simulink model "single_phase_multilevel"  (R2023b)
settings: Solver=ode1be  StartTime=0.0  StopTime=simlength  FixedStep=tc  RelTol=1e-3
values from neighbouring files (symbols this model uses):
  Vfc1_base = Udc/5    [plotting_modulation.m]
  Vfc2_base = 2*Vfc1_base    [plotting_modulation.m]
  Vfc3_base = 3*Vfc1_base    [plotting_modulation.m]
  Vfc4_base = 4*Vfc1_base    [plotting_modulation.m]
undefined symbols (not defined in the file or in its folder): __PRM__SERIALIZED__DATA__, DThs_init, g0_4Hz, g1_4Hz, I_FS, kalman_omega, kalman_theta, ki_i_inv, ki_v_inv, kp_i_inv, kp_v_inv, Lconn, LFu1, m_dead_time, m_duty_open_loop, magnitude, n10, omega_ref, phase_shift_mod11, phase_shift_mod21, phase_shift_mod31, phase_shift_mod41, phase_shift_mod51, precharge_off, q1kalman, q2kalman, Rbalance, Rconn, RFu, Rg_off, Rg_on, Rkalman, RLFu1, Rprecharge, Tambient, tc, time_pwm_enable, tPWM, ts, V_FS, VCFc_5_init, Vgate_base, weigth
libraries: fl_lib x271, nesl_utility x97, ee_lib x15, simulink x1
(part 4 of 5)

== system single_phase_multilevel/flying_capacitor_leg/switch_51 ==
  G : Inport
  Current Sensor : fl_lib/Electrical/Electrical Sensors/Current Sensor
  Electrical Reference : fl_lib/Electrical/Electrical Elements/Electrical Reference
  G3R160MT17D : ee_lib/Semiconductors & Converters/MOSFET (Ideal, Switching)  port_option=ee.enum.controlport.elec  Rds=Rds_on Ohm  Goff=Goff_state_mosfet 1/Ohm  Vth=Vg_threshold V  diode_param=ee.enum.converters.protectiondiode.nodynamics  diode_Vf=Vgamma_diode_mosfet V  diode_Ron=Ron_diode_mosfet Ohm  diode_Goff=Goff_state_mosfet 1/Ohm  diode_C=50e-9 F  diode_iRM=-235 A  diode_iF=300 A  diode_idot=-50 A/us  diode_trr_param=ee.enum.converters.diodeReverseParam.trr_factor  diode_trr_factor=3  diode_trr=15 us  diode_Qrr=1500 s*uA  ids_specify=off  ids_priority=None  ids=0 A  ids_nominal_specify=off  ids_nominal_unit=A  ids_nominal_value=1  vds_specify=off  vds_priority=None  vds=0 V  vds_nominal_specify=off  vds_nominal_unit=V  vds_nominal_value=1  vgs_specify=off  vgs_priority=None  vgs=0 V  vgs_nominal_specify=off  vgs_nominal_unit=V  vgs_nominal_value=1  thermal_loss_option=ee.enum.converters.thermalLossOption.constantvalues  Von_data=[0, 1.8, 3.2, 6, 10, 16; 0, 2, 5.5, 9.5, 15, 25] V  Tj=[298.15, 448.15] K  Iout_data=[0, 20, 40, 60, 80, 100] A  Eon_data=[0, 55.04, 124.57, 235.53, 362.12; 0, 71.25, 161.25, 304.88, 468.75] * 1e-6 J  Eoff_data=[0, 18, 30, 56.1, 76.5; 0, 22.5, 37.5, 70.13, 95.63] * 1e-6 J  Eon_data_3D=[zeros(2, 5, 3)] J  Eoff_data_3D=[zeros(2, 5, 3)] J  Tj_loss=[298.15, 448.15] K  Iout_data_loss=[0, 10, 20, 30, 40] A  tabulateWithVds=false  Vds_loss=[0, 150, 300] V  Eon_scalar=Eon J  Eoff_scalar=Eoff J  Voff=Vdc_switching_losses_ref V  Iout_scalar=Ids_switching_losses_ref A  useCurrentFromPreviousCycle=true  useVoltageFromPreviousCycle=true  diodeModelType=ee.enum.converters.diodeModelType.pwl  diodeTableType=ee.enum.diode.tableType.IfMat  diode_IfMat=[.07, .12, .19, 1.75, 4.24, 7.32, 11.2; .16, .3, .72, 2.14, 4.02, 6.35, 9.12] A  diode_VfMat=[.9, 1.15, 1.25, 1.5, 1.75, 2.17, 2.6, 2.85; .58, .68, .75, 1.1, 1.38, 1.77, 2.27, 2.7] V  diode_TjVec=[25, 125] degC  diode_VfVec=[.5, .7, .9, 1.3, 1.7, 2.1, 2.5] V  diode_IfVec=[.1, .2, .5, 1, 2, 4, 7, 10] A  diode_Vr=-600 V  diode_Ls=150 nH  diode_Erec=0.03 J  diode_rec_loss_model=ee.enum.diode.reverseRecoveryModel.fixed  diode_ErecVal=0 J  diode_scaleWithIandV=true  diode_ErecMat=zeros(2, 3) J  diode_TjrecVec=[298.15, 398.15] K  diode_IfrecVec=[.1, 1, 10] A  diode_IrecVal=10 A  diode_VrecVal=10 V  diode_tFilter=1 / 1000 / 100 s  thermal_network_parameterization=ee.enum.thermalNetworkTopology.external  Rth=[.03, .2] K/W  Rth_Cauer=[.03, .1, .2] K/W  Rth_Foster=[.03, .2] K/W  thermal_mass_parameterization=ee.enum.thermalNetwork.timeconstant  thermal_mass=[3, 25] J/K  thermal_mass_Cauer=[3, 10, 25] J/K  thermal_mass_Foster=[33, 50] J/K  thermal_time_constant=[.1, 5] s  thermal_time_constant_Cauer=[.1, 1, 5] s  thermal_time_constant_Foster=[1, 10] s  thermal_mass_initial_temperatures=[25, 25] degC  thermal_mass_initial_temperatures_Cauer=[25, 25, 25] degC  junction_thermal_mass=JunctionTermalMass J/K  Tvec_initial_Foster=[25, 25, 25, 25] degC  no_thermal_network=0  junction_temperature_specify=off  junction_temperature_priority=None  junction_temperature=25 degC  junction_temperature_nominal_specify=off  junction_temperature_nominal_unit=degC  junction_temperature_nominal_value=1  Qj_specify=off  Qj_priority=None  Qj=0 W  Qj_nominal_specify=off  Qj_nominal_unit=W  Qj_nominal_value=1  accumulatedSwitchingLosses_specify=off  accumulatedSwitchingLosses_priority=None  accumulatedSwitchingLosses=0 J
      settings: InternalSimscapePortConfiguration="{\"Bottom\":[],\"Left\":[{\"id\":\"G_elec\",\"label\":\"\",\"type\":\"foundation.electrical.electrical\"},{\"id\":\"H\",\"label\":\"\",\"type\":\"foundation.thermal.thermal\"}],\"Right\":[{\"id\":\"D\",\"label\":\"\",\"type\":\"foundation.electrical.electrical\"},{\"id\":\"S\",\"label\":\"\",\"type\":\"foundation.electrical.electrical\"}],\"Top\":[]}"
  Heat Flow Rate Sensor : fl_lib/Thermal/Thermal Sensors/Heat Flow Rate Sensor
  Lstray : fl_lib/Electrical/Electrical Elements/Inductor  l=Lstray H  r=0 Ohm  g=1e-9 1/Ohm  i_specify=off  i_priority=None  i=0 A  i_nominal_specify=off  i_nominal_unit=A  i_nominal_value=1  v_specify=off  v_priority=None  v=0 V  v_nominal_specify=off  v_nominal_unit=V  v_nominal_value=1  i_L_specify=off  i_L_priority=High  i_L=0 A  i_L_nominal_specify=off  i_L_nominal_unit=A  i_L_nominal_value=1
  Mux : Mux  Inputs=2
  PS-Simulink Converter : nesl_utility/PS-Simulink Converter  PhysicalDomain=network_engine_domain  SubClassName=ps_output  LeftPortType=input  RightPortType=output  PseudoPeriodic=off  Frequencies=[]  VectorFormat=1-D array  Unit=W  AffineConversion=off
  PS-Simulink Converter1 : nesl_utility/PS-Simulink Converter  PhysicalDomain=network_engine_domain  SubClassName=ps_output  LeftPortType=input  RightPortType=output  PseudoPeriodic=off  Frequencies=[]  VectorFormat=1-D array  Unit=V  AffineConversion=off
  PS-Simulink Converter2 : nesl_utility/PS-Simulink Converter  PhysicalDomain=network_engine_domain  SubClassName=ps_output  LeftPortType=input  RightPortType=output  PseudoPeriodic=off  Frequencies=[]  VectorFormat=1-D array  Unit=degC  AffineConversion=off
  PS-Simulink Converter3 : nesl_utility/PS-Simulink Converter  PhysicalDomain=network_engine_domain  SubClassName=ps_output  LeftPortType=input  RightPortType=output  PseudoPeriodic=off  Frequencies=[]  VectorFormat=1-D array  Unit=degC  AffineConversion=off
  PS-Simulink Converter4 : nesl_utility/PS-Simulink Converter  PhysicalDomain=network_engine_domain  SubClassName=ps_output  LeftPortType=input  RightPortType=output  PseudoPeriodic=off  Frequencies=[]  VectorFormat=1-D array  Unit=A  AffineConversion=off
  PS-Simulink Converter5 : nesl_utility/PS-Simulink Converter  PhysicalDomain=network_engine_domain  SubClassName=ps_output  LeftPortType=input  RightPortType=output  PseudoPeriodic=off  Frequencies=[]  VectorFormat=1-D array  Unit=V  AffineConversion=off
  Tambient : fl_lib/Thermal/Thermal Sources/Temperature Source  temperature=Tambient degC
  Temperature Sensor : fl_lib/Thermal/Thermal Sensors/Temperature Sensor  temperature_measure=foundation.enum.MeasurementReference.difference
  Temperature Sensor1 : fl_lib/Thermal/Thermal Sensors/Temperature Sensor  temperature_measure=foundation.enum.MeasurementReference.difference
  Voltage Sensor : fl_lib/Electrical/Electrical Sensors/Voltage Sensor
  Voltage Sensor1 : fl_lib/Electrical/Electrical Sensors/Voltage Sensor
  gate_driver : Subsystem
  heatsink_C : fl_lib/Thermal/Thermal Elements/Thermal Mass  Commented=on  mass_type=foundation.enum.constant_variable.constant  mass=weigth/6 kg  sp_heat=cp_al J/(K*kg)  mass_min=1e-6 kg  num_ports=foundation.enum.numPorts2.one  m_specify=off  m_priority=High  m=1 kg  m_nominal_specify=off  m_nominal_unit=kg  m_nominal_value=1  T_specify=on  T_priority=High  T=DThs_init+Tambient degC  T_nominal_specify=off  T_nominal_unit=K  T_nominal_value=1  Q_specify=off  Q_priority=High  Q=0 W  Q_nominal_specify=off  Q_nominal_unit=W  Q_nominal_value=1
  heatsink_R : fl_lib/Thermal/Thermal Elements/Thermal Resistance  resistance=Rth_mosfet_HA K/W  T_specify=off  T_priority=High  T=0 deltadegC  T_nominal_specify=off  T_nominal_unit=K  T_nominal_value=1  Q_specify=off  Q_priority=None  Q=0 W  Q_nominal_specify=off  Q_nominal_unit=W  Q_nominal_value=1
  mosfet_sandwich : fl_lib/Thermal/Thermal Elements/Thermal Resistance  resistance=Rth_mosfet_JH K/W  T_specify=off  T_priority=High  T=0 degC  T_nominal_specify=off  T_nominal_unit=K  T_nominal_value=1  Q_specify=off  Q_priority=None  Q=0 W  Q_nominal_specify=off  Q_nominal_unit=W  Q_nominal_value=1
  power_losses_mosfet : Scope  Commented=on  NumInputPorts=2
  D : PMIOPort  Side=Left
  S : PMIOPort  Port=2  Side=Right
  tag scope: device_current_51=global, device_voltage_51=global, mosfet_51_power_losses=global, temperature_mosfet_51_HA=global, temperature_mosfet_51_JH=global, voltage_cm_device_51=global
  wires:
  PS-Simulink Converter1/1 -> [device_voltage_51]
  Mux/1 -> power_losses_mosfet/2
  PS-Simulink Converter3/1 -> [temperature_mosfet_51_HA]  "mosfet_HA_temp"
  [temperature_mosfet_51_JH] -> Mux/1
  [temperature_mosfet_51_HA] -> Mux/2
  PS-Simulink Converter2/1 -> [temperature_mosfet_51_JH]  "mosfet_JH_temp"
  PS-Simulink Converter/1 -> power_losses_mosfet/1, [mosfet_51_power_losses]  "Power Losses"
  PS-Simulink Converter4/1 -> [device_current_51]
  PS-Simulink Converter5/1 -> [voltage_cm_device_51]
  G/1 -> gate_driver/1(cmd)
  connections:
  Voltage Sensor/RConn1 -- PS-Simulink Converter1/LConn1
  mosfet_sandwich/LConn1 -- Temperature Sensor/LConn1 -- Heat Flow Rate Sensor/RConn2
  heatsink_R/RConn1 -- Tambient/LConn1 -- Temperature Sensor1/RConn1
  heatsink_C/LConn1 -- mosfet_sandwich/RConn1 -- Temperature Sensor1/LConn1 -- Temperature Sensor/RConn1 -- heatsink_R/LConn1
  Temperature Sensor1/RConn2 -- PS-Simulink Converter3/LConn1
  D/RConn1 -- Current Sensor/LConn1 -- Voltage Sensor/LConn1
  Temperature Sensor/RConn2 -- PS-Simulink Converter2/LConn1
  Voltage Sensor/RConn2 -- S/RConn1 -- gate_driver/RConn2 -- G3R160MT17D/RConn2 -- Voltage Sensor1/LConn1
  PS-Simulink Converter/LConn1 -- Heat Flow Rate Sensor/RConn1
  G3R160MT17D/LConn2 -- Heat Flow Rate Sensor/LConn1
  G3R160MT17D/RConn1 -- Lstray/RConn1
  Current Sensor/RConn1 -- PS-Simulink Converter4/LConn1
  Voltage Sensor1/RConn2 -- Electrical Reference/LConn1
  PS-Simulink Converter5/LConn1 -- Voltage Sensor1/RConn1
  Lstray/LConn1 -- Current Sensor/RConn2
  gate_driver/RConn1 -- G3R160MT17D/LConn1

== system single_phase_multilevel/flying_capacitor_leg/switch_52 ==
  G : Inport
  Current Sensor : fl_lib/Electrical/Electrical Sensors/Current Sensor
  Electrical Reference : fl_lib/Electrical/Electrical Elements/Electrical Reference
  G3R160MT17D : ee_lib/Semiconductors & Converters/MOSFET (Ideal, Switching)  port_option=ee.enum.controlport.elec  Rds=Rds_on Ohm  Goff=Goff_state_mosfet 1/Ohm  Vth=Vg_threshold V  diode_param=ee.enum.converters.protectiondiode.nodynamics  diode_Vf=Vgamma_diode_mosfet V  diode_Ron=Ron_diode_mosfet Ohm  diode_Goff=Goff_state_mosfet 1/Ohm  diode_C=50e-9 F  diode_iRM=-235 A  diode_iF=300 A  diode_idot=-50 A/us  diode_trr_param=ee.enum.converters.diodeReverseParam.trr_factor  diode_trr_factor=3  diode_trr=15 us  diode_Qrr=1500 s*uA  ids_specify=off  ids_priority=None  ids=0 A  ids_nominal_specify=off  ids_nominal_unit=A  ids_nominal_value=1  vds_specify=off  vds_priority=None  vds=0 V  vds_nominal_specify=off  vds_nominal_unit=V  vds_nominal_value=1  vgs_specify=off  vgs_priority=None  vgs=0 V  vgs_nominal_specify=off  vgs_nominal_unit=V  vgs_nominal_value=1  thermal_loss_option=ee.enum.converters.thermalLossOption.constantvalues  Von_data=[0, 1.8, 3.2, 6, 10, 16; 0, 2, 5.5, 9.5, 15, 25] V  Tj=[298.15, 448.15] K  Iout_data=[0, 20, 40, 60, 80, 100] A  Eon_data=[0, 55.04, 124.57, 235.53, 362.12; 0, 71.25, 161.25, 304.88, 468.75] * 1e-6 J  Eoff_data=[0, 18, 30, 56.1, 76.5; 0, 22.5, 37.5, 70.13, 95.63] * 1e-6 J  Eon_data_3D=[zeros(2, 5, 3)] J  Eoff_data_3D=[zeros(2, 5, 3)] J  Tj_loss=[298.15, 448.15] K  Iout_data_loss=[0, 10, 20, 30, 40] A  tabulateWithVds=false  Vds_loss=[0, 150, 300] V  Eon_scalar=Eon J  Eoff_scalar=Eoff J  Voff=Vdc_switching_losses_ref V  Iout_scalar=Ids_switching_losses_ref A  useCurrentFromPreviousCycle=true  useVoltageFromPreviousCycle=true  diodeModelType=ee.enum.converters.diodeModelType.pwl  diodeTableType=ee.enum.diode.tableType.IfMat  diode_IfMat=[.07, .12, .19, 1.75, 4.24, 7.32, 11.2; .16, .3, .72, 2.14, 4.02, 6.35, 9.12] A  diode_VfMat=[.9, 1.15, 1.25, 1.5, 1.75, 2.17, 2.6, 2.85; .58, .68, .75, 1.1, 1.38, 1.77, 2.27, 2.7] V  diode_TjVec=[25, 125] degC  diode_VfVec=[.5, .7, .9, 1.3, 1.7, 2.1, 2.5] V  diode_IfVec=[.1, .2, .5, 1, 2, 4, 7, 10] A  diode_Vr=-600 V  diode_Ls=150 nH  diode_Erec=0.03 J  diode_rec_loss_model=ee.enum.diode.reverseRecoveryModel.fixed  diode_ErecVal=0 J  diode_scaleWithIandV=true  diode_ErecMat=zeros(2, 3) J  diode_TjrecVec=[298.15, 398.15] K  diode_IfrecVec=[.1, 1, 10] A  diode_IrecVal=10 A  diode_VrecVal=10 V  diode_tFilter=1 / 1000 / 100 s  thermal_network_parameterization=ee.enum.thermalNetworkTopology.external  Rth=[.03, .2] K/W  Rth_Cauer=[.03, .1, .2] K/W  Rth_Foster=[.03, .2] K/W  thermal_mass_parameterization=ee.enum.thermalNetwork.timeconstant  thermal_mass=[3, 25] J/K  thermal_mass_Cauer=[3, 10, 25] J/K  thermal_mass_Foster=[33, 50] J/K  thermal_time_constant=[.1, 5] s  thermal_time_constant_Cauer=[.1, 1, 5] s  thermal_time_constant_Foster=[1, 10] s  thermal_mass_initial_temperatures=[25, 25] degC  thermal_mass_initial_temperatures_Cauer=[25, 25, 25] degC  junction_thermal_mass=JunctionTermalMass J/K  Tvec_initial_Foster=[25, 25, 25, 25] degC  no_thermal_network=0  junction_temperature_specify=off  junction_temperature_priority=None  junction_temperature=25 degC  junction_temperature_nominal_specify=off  junction_temperature_nominal_unit=degC  junction_temperature_nominal_value=1  Qj_specify=off  Qj_priority=None  Qj=0 W  Qj_nominal_specify=off  Qj_nominal_unit=W  Qj_nominal_value=1  accumulatedSwitchingLosses_specify=off  accumulatedSwitchingLosses_priority=None  accumulatedSwitchingLosses=0 J
      settings: InternalSimscapePortConfiguration="{\"Bottom\":[],\"Left\":[{\"id\":\"G_elec\",\"label\":\"\",\"type\":\"foundation.electrical.electrical\"},{\"id\":\"H\",\"label\":\"\",\"type\":\"foundation.thermal.thermal\"}],\"Right\":[{\"id\":\"D\",\"label\":\"\",\"type\":\"foundation.electrical.electrical\"},{\"id\":\"S\",\"label\":\"\",\"type\":\"foundation.electrical.electrical\"}],\"Top\":[]}"
  Heat Flow Rate Sensor : fl_lib/Thermal/Thermal Sensors/Heat Flow Rate Sensor
  Lstray : fl_lib/Electrical/Electrical Elements/Inductor  l=Lstray H  r=0 Ohm  g=1e-9 1/Ohm  i_specify=off  i_priority=None  i=0 A  i_nominal_specify=off  i_nominal_unit=A  i_nominal_value=1  v_specify=off  v_priority=None  v=0 V  v_nominal_specify=off  v_nominal_unit=V  v_nominal_value=1  i_L_specify=off  i_L_priority=High  i_L=0 A  i_L_nominal_specify=off  i_L_nominal_unit=A  i_L_nominal_value=1
  Mux : Mux  Inputs=2
  PS-Simulink Converter : nesl_utility/PS-Simulink Converter  PhysicalDomain=network_engine_domain  SubClassName=ps_output  LeftPortType=input  RightPortType=output  PseudoPeriodic=off  Frequencies=[]  VectorFormat=1-D array  Unit=W  AffineConversion=off
  PS-Simulink Converter1 : nesl_utility/PS-Simulink Converter  PhysicalDomain=network_engine_domain  SubClassName=ps_output  LeftPortType=input  RightPortType=output  PseudoPeriodic=off  Frequencies=[]  VectorFormat=1-D array  Unit=V  AffineConversion=off
  PS-Simulink Converter2 : nesl_utility/PS-Simulink Converter  PhysicalDomain=network_engine_domain  SubClassName=ps_output  LeftPortType=input  RightPortType=output  PseudoPeriodic=off  Frequencies=[]  VectorFormat=1-D array  Unit=degC  AffineConversion=off
  PS-Simulink Converter3 : nesl_utility/PS-Simulink Converter  PhysicalDomain=network_engine_domain  SubClassName=ps_output  LeftPortType=input  RightPortType=output  PseudoPeriodic=off  Frequencies=[]  VectorFormat=1-D array  Unit=degC  AffineConversion=off
  PS-Simulink Converter4 : nesl_utility/PS-Simulink Converter  PhysicalDomain=network_engine_domain  SubClassName=ps_output  LeftPortType=input  RightPortType=output  PseudoPeriodic=off  Frequencies=[]  VectorFormat=1-D array  Unit=A  AffineConversion=off
  PS-Simulink Converter5 : nesl_utility/PS-Simulink Converter  PhysicalDomain=network_engine_domain  SubClassName=ps_output  LeftPortType=input  RightPortType=output  PseudoPeriodic=off  Frequencies=[]  VectorFormat=1-D array  Unit=V  AffineConversion=off
  Tambient : fl_lib/Thermal/Thermal Sources/Temperature Source  temperature=Tambient degC
  Temperature Sensor : fl_lib/Thermal/Thermal Sensors/Temperature Sensor  temperature_measure=foundation.enum.MeasurementReference.difference
  Temperature Sensor1 : fl_lib/Thermal/Thermal Sensors/Temperature Sensor  temperature_measure=foundation.enum.MeasurementReference.difference
  Voltage Sensor : fl_lib/Electrical/Electrical Sensors/Voltage Sensor
  Voltage Sensor1 : fl_lib/Electrical/Electrical Sensors/Voltage Sensor
  gate_driver : Subsystem
  heatsink_C : fl_lib/Thermal/Thermal Elements/Thermal Mass  Commented=on  mass_type=foundation.enum.constant_variable.constant  mass=weigth/6 kg  sp_heat=cp_al J/(K*kg)  mass_min=1e-6 kg  num_ports=foundation.enum.numPorts2.one  m_specify=off  m_priority=High  m=1 kg  m_nominal_specify=off  m_nominal_unit=kg  m_nominal_value=1  T_specify=on  T_priority=High  T=DThs_init+Tambient degC  T_nominal_specify=off  T_nominal_unit=K  T_nominal_value=1  Q_specify=off  Q_priority=High  Q=0 W  Q_nominal_specify=off  Q_nominal_unit=W  Q_nominal_value=1
  heatsink_R : fl_lib/Thermal/Thermal Elements/Thermal Resistance  resistance=Rth_mosfet_HA K/W  T_specify=off  T_priority=High  T=0 deltadegC  T_nominal_specify=off  T_nominal_unit=K  T_nominal_value=1  Q_specify=off  Q_priority=None  Q=0 W  Q_nominal_specify=off  Q_nominal_unit=W  Q_nominal_value=1
  mosfet_sandwich : fl_lib/Thermal/Thermal Elements/Thermal Resistance  resistance=Rth_mosfet_JH K/W  T_specify=off  T_priority=High  T=0 degC  T_nominal_specify=off  T_nominal_unit=K  T_nominal_value=1  Q_specify=off  Q_priority=None  Q=0 W  Q_nominal_specify=off  Q_nominal_unit=W  Q_nominal_value=1
  power_losses_mosfet : Scope  Commented=on  NumInputPorts=2
  D : PMIOPort  Side=Left
  S : PMIOPort  Port=2  Side=Right
  tag scope: device_current_52=global, device_voltage_52=global, mosfet_52_power_losses=global, temperature_mosfet_52_HA=global, temperature_mosfet_52_JH=global, voltage_cm_device_52=global
  wires:
  PS-Simulink Converter/1 -> [mosfet_52_power_losses], power_losses_mosfet/1  "Power Losses"
  PS-Simulink Converter2/1 -> [temperature_mosfet_52_JH]  "mosfet_JH_temp"
  [temperature_mosfet_52_HA] -> Mux/2
  [temperature_mosfet_52_JH] -> Mux/1
  PS-Simulink Converter3/1 -> [temperature_mosfet_52_HA]  "mosfet_HA_temp"
  Mux/1 -> power_losses_mosfet/2
  PS-Simulink Converter1/1 -> [device_voltage_52]
  PS-Simulink Converter4/1 -> [device_current_52]
  PS-Simulink Converter5/1 -> [voltage_cm_device_52]
  G/1 -> gate_driver/1(cmd)
  connections:
  G3R160MT17D/LConn2 -- Heat Flow Rate Sensor/LConn1
  PS-Simulink Converter/LConn1 -- Heat Flow Rate Sensor/RConn1
  Voltage Sensor/RConn2 -- gate_driver/RConn2 -- S/RConn1 -- G3R160MT17D/RConn2 -- Voltage Sensor1/LConn1
  Temperature Sensor/RConn2 -- PS-Simulink Converter2/LConn1
  Temperature Sensor1/RConn2 -- PS-Simulink Converter3/LConn1
  mosfet_sandwich/RConn1 -- heatsink_C/LConn1 -- heatsink_R/LConn1 -- Temperature Sensor/RConn1 -- Temperature Sensor1/LConn1
  Tambient/LConn1 -- heatsink_R/RConn1 -- Temperature Sensor1/RConn1
  Temperature Sensor/LConn1 -- mosfet_sandwich/LConn1 -- Heat Flow Rate Sensor/RConn2
  Voltage Sensor/RConn1 -- PS-Simulink Converter1/LConn1
  Current Sensor/LConn1 -- D/RConn1 -- Voltage Sensor/LConn1
  G3R160MT17D/RConn1 -- Lstray/RConn1
  Current Sensor/RConn1 -- PS-Simulink Converter4/LConn1
  PS-Simulink Converter5/LConn1 -- Voltage Sensor1/RConn1
  Voltage Sensor1/RConn2 -- Electrical Reference/LConn1
  Lstray/LConn1 -- Current Sensor/RConn2
  G3R160MT17D/LConn1 -- gate_driver/RConn1

== system single_phase_multilevel/flying_capacitor_leg/vm ==
  CFi_HF_5 : fl_lib/Electrical/Electrical Elements/Capacitor  c=CFi_HF_5 F  r=1e-6 Ohm  g=0 1/Ohm  i_specify=off  i_priority=None  i=0 A  i_nominal_specify=off  i_nominal_unit=A  i_nominal_value=1  v_specify=off  v_priority=None  v=0 V  v_nominal_specify=off  v_nominal_unit=V  v_nominal_value=1  vc_specify=on  vc_priority=High  vc=VCFc_5_init V  vc_nominal_specify=off  vc_nominal_unit=V  vc_nominal_value=1
  LCFi_HF_5 : fl_lib/Electrical/Electrical Elements/Inductor  l=LCFi_HF_5 H  r=RCFi_HF_5 Ohm  g=1e-9 1/Ohm  i_specify=off  i_priority=None  i=0 A  i_nominal_specify=off  i_nominal_unit=A  i_nominal_value=1  v_specify=off  v_priority=None  v=0 V  v_nominal_specify=off  v_nominal_unit=V  v_nominal_value=1  i_L_specify=off  i_L_priority=High  i_L=0 A  i_L_nominal_specify=off  i_L_nominal_unit=A  i_L_nominal_value=1
  PS-Simulink Converter2 : nesl_utility/PS-Simulink Converter  PhysicalDomain=network_engine_domain  SubClassName=ps_output  LeftPortType=input  RightPortType=output  PseudoPeriodic=off  Frequencies=[]  VectorFormat=1-D array  Unit=V  AffineConversion=off
  Voltage Sensor1 : fl_lib/Electrical/Electrical Sensors/Voltage Sensor
  1 : PMIOPort  Side=Left
  2 : PMIOPort  Port=2  Side=Right
  tag scope: voltage_flying_capacitor_5=global
  wires:
  PS-Simulink Converter2/1 -> [voltage_flying_capacitor_5]
  connections:
  Voltage Sensor1/RConn2 -- LCFi_HF_5/RConn1 -- 2/RConn1
  Voltage Sensor1/RConn1 -- PS-Simulink Converter2/LConn1
  Voltage Sensor1/LConn1 -- CFi_HF_5/LConn1 -- 1/RConn1
  LCFi_HF_5/LConn1 -- CFi_HF_5/RConn1

== system single_phase_multilevel/output_filter/Subsystem ==
  PS Step1 : fl_lib/Physical Signals/Sources/PS Step  step_time=load_on s  initial_value=0  final_value=1
  Switch1 : fl_lib/Electrical/Electrical Elements/Switch  R_closed=0.01 Ohm  G_open=1e-8 1/Ohm  Threshold=0.5  i_specify=off  i_priority=None  i=0 A  i_nominal_specify=off  i_nominal_unit=A  i_nominal_value=1  v_specify=off  v_priority=None  v=0 V  v_nominal_specify=off  v_nominal_unit=V  v_nominal_value=1
  Variant Connector : VariantPMConnector  VariantControls=__PRM__SERIALIZED__DATA__:  ConnectorBlkType=Nonprimary
  Variant Connector1 : VariantPMConnector  VariantControls=__PRM__SERIALIZED__DATA__:enable_dclink_precharge == 1  ConnectorBlkType=Primary  ConnectorTag=B  ShowConditionOnBlock=on
  Variant Connector2 : VariantPMConnector  VariantControls=__PRM__SERIALIZED__DATA__:enable_dclink_precharge == 0  ConnectorBlkType=Primary  ShowConditionOnBlock=on
  Variant Connector3 : VariantPMConnector  VariantControls=__PRM__SERIALIZED__DATA__:  ConnectorBlkType=Nonprimary  ConnectorTag=B
  Conn1 : PMIOPort  Side=Left
  Conn2 : PMIOPort  Port=2  Side=Right
  connections:
  Variant Connector1/LConn1 -- Switch1/RConn2
  PS Step1/RConn1 -- Switch1/RConn1
  Conn1/RConn1 -- Variant Connector3/RConn1 -- Variant Connector/RConn1
  Variant Connector/LConn1 -- Variant Connector2/LConn1
  Conn2/RConn1 -- Variant Connector2/RConn1 -- Variant Connector1/RConn1
  Switch1/LConn1 -- Variant Connector3/LConn1

== system single_phase_multilevel/output_filter/instantaneus_power ==
  vout : Inport
  iout : Inport  Port=2
  Product : Product
  To Workspace3 : ToWorkspace  VariableName=vout_rms_sim  SampleTime=ts
      settings: MaxDataPoints=Ns
  To Workspace4 : ToWorkspace  VariableName=iout_rms_sim  SampleTime=ts
      settings: MaxDataPoints=Ns
  To Workspace7 : ToWorkspace  VariableName=Pout_avg_sim  SampleTime=ts
      settings: MaxDataPoints=Ns
  moving_avarage : Subsystem
  rms&power : Scope  NumInputPorts=3
  rms2 : Subsystem
  rms3 : Subsystem
  tag scope: inverter_current_output=global, inverter_voltage_output=global
  wires:
  rms2/1(Out1) -> rms&power/1, To Workspace3/1  "vout_rms"
  rms3/1(Out1) -> rms&power/3, To Workspace4/1  "iout_rms"
  vout/1 -> [inverter_voltage_output], rms2/1(vout), Product/1
  iout/1 -> [inverter_current_output], rms3/1(iout), Product/2
  Product/1 -> moving_avarage/1(In)
  moving_avarage/1(Mean) -> rms&power/2, To Workspace7/1  "pout_mean"

== system single_phase_multilevel/output_filter/voltage_measure ==
  C1_100n : fl_lib/Electrical/Electrical Elements/Capacitor  Commented=on  c=100e-9 F  r=1e-6 Ohm  g=0 1/Ohm  i_specify=off  i_priority=None  i=0 A  i_nominal_specify=off  i_nominal_unit=A  i_nominal_value=1  v_specify=off  v_priority=None  v=0 V  v_nominal_specify=off  v_nominal_unit=V  v_nominal_value=1  vc_specify=off  vc_priority=High  vc=0 V  vc_nominal_specify=off  vc_nominal_unit=V  vc_nominal_value=1
  C2_100n : fl_lib/Electrical/Electrical Elements/Capacitor  Commented=on  c=100e-9 F  r=1e-6 Ohm  g=0 1/Ohm  i_specify=off  i_priority=None  i=0 A  i_nominal_specify=off  i_nominal_unit=A  i_nominal_value=1  v_specify=off  v_priority=None  v=0 V  v_nominal_specify=off  v_nominal_unit=V  v_nominal_value=1  vc_specify=off  vc_priority=High  vc=0 V  vc_nominal_specify=off  vc_nominal_unit=V  vc_nominal_value=1
  C3_100n : fl_lib/Electrical/Electrical Elements/Capacitor  c=100e-9 F  r=1e-6 Ohm  g=0 1/Ohm  i_specify=off  i_priority=None  i=0 A  i_nominal_specify=off  i_nominal_unit=A  i_nominal_value=1  v_specify=off  v_priority=None  v=0 V  v_nominal_specify=off  v_nominal_unit=V  v_nominal_value=1  vc_specify=off  vc_priority=High  vc=0 V  vc_nominal_specify=off  vc_nominal_unit=V  vc_nominal_value=1
  R1_49k5 : fl_lib/Electrical/Electrical Elements/Resistor  R=49.5e3 Ohm  i_specify=off  i_priority=None  i=0 A  i_nominal_specify=off  i_nominal_unit=A  i_nominal_value=1  v_specify=off  v_priority=None  v=0 V  v_nominal_specify=off  v_nominal_unit=V  v_nominal_value=1
  R2_49k5 : fl_lib/Electrical/Electrical Elements/Resistor  R=49.5e3 Ohm  i_specify=off  i_priority=None  i=0 A  i_nominal_specify=off  i_nominal_unit=A  i_nominal_value=1  v_specify=off  v_priority=None  v=0 V  v_nominal_specify=off  v_nominal_unit=V  v_nominal_value=1
  R3_225 : fl_lib/Electrical/Electrical Elements/Resistor  R=225 Ohm  i_specify=off  i_priority=None  i=0 A  i_nominal_specify=off  i_nominal_unit=A  i_nominal_value=1  v_specify=off  v_priority=None  v=0 V  v_nominal_specify=off  v_nominal_unit=V  v_nominal_value=1
  R4_5k : fl_lib/Electrical/Electrical Elements/Resistor  R=5e3 Ohm  i_specify=off  i_priority=None  i=0 A  i_nominal_specify=off  i_nominal_unit=A  i_nominal_value=1  v_specify=off  v_priority=None  v=0 V  v_nominal_specify=off  v_nominal_unit=V  v_nominal_value=1
  R5_5k : fl_lib/Electrical/Electrical Elements/Resistor  R=5e3 Ohm  i_specify=off  i_priority=None  i=0 A  i_nominal_specify=off  i_nominal_unit=A  i_nominal_value=1  v_specify=off  v_priority=None  v=0 V  v_nominal_specify=off  v_nominal_unit=V  v_nominal_value=1
  voltage_measure : Subsystem
  U(+) : PMIOPort  Side=Right
  U(-) : PMIOPort  Port=2  Side=Right
  connections:
  U(+)/RConn1 -- R1_49k5/LConn1 -- C1_100n/LConn1
  R2_49k5/RConn1 -- C2_100n/RConn1 -- U(-)/RConn1
  R3_225/LConn1 -- R1_49k5/RConn1 -- C3_100n/LConn1 -- C1_100n/RConn1 -- R4_5k/RConn1
  R3_225/RConn1 -- C2_100n/LConn1 -- C3_100n/RConn1 -- R5_5k/RConn1 -- R2_49k5/LConn1
  voltage_measure/LConn1 -- R4_5k/LConn1
  voltage_measure/LConn2 -- R5_5k/LConn1

== system single_phase_multilevel/vi_ctrl/modulator1 ==
  m : Inport
  Constant7 : Constant  Value=-m_dead_time
  Constant8 : Constant  Value=m_dead_time
  Data Type Conversion : DataTypeConversion  OutDataTypeStr=double  SaturateOnIntegerOverflow=off  RndMeth=Floor
  Data Type Conversion1 : DataTypeConversion  OutDataTypeStr=double  SaturateOnIntegerOverflow=off  RndMeth=Floor
  Gain : Gain  Gain=Vgate_base
  Gain1 : Gain  Gain=Vgate_base
  Relational Operator : RelationalOperator  Operator=<=
  Relational Operator1 : RelationalOperator  Operator=<=
  Sum1 : Sum  Inputs=|++
  Sum2 : Sum  Inputs=++|
  g11/g12 : Scope  NumInputPorts=2
  triangle_1 : Subsystem
  g11 : Outport
  g12 : Outport  Port=2
  tag scope: carry_g11=global
  wires:
  m/1 -> Sum1/2, Sum2/1
  Relational Operator/1 -> Data Type Conversion/1
  Relational Operator1/1 -> Data Type Conversion1/1
  Data Type Conversion/1 -> g11/g12/1, Gain/1
  triangle_1/1(carry_mod11) -> Relational Operator1/2, Relational Operator/1, [carry_g11]
  Constant7/1 -> Sum1/1
  Data Type Conversion1/1 -> g11/g12/2, Gain1/1
  Sum2/1 -> Relational Operator1/1
  Constant8/1 -> Sum2/2
  Sum1/1 -> Relational Operator/2
  Gain/1 -> g11/1
  Gain1/1 -> g12/1

== system single_phase_multilevel/vi_ctrl/modulator2 ==
  m : Inport
  Constant7 : Constant  Value=-m_dead_time
  Constant8 : Constant  Value=m_dead_time
  Data Type Conversion : DataTypeConversion  OutDataTypeStr=double  SaturateOnIntegerOverflow=off  RndMeth=Floor
  Data Type Conversion1 : DataTypeConversion  OutDataTypeStr=double  SaturateOnIntegerOverflow=off  RndMeth=Floor
  Gain : Gain  Gain=Vgate_base
  Gain1 : Gain  Gain=Vgate_base
  Relational Operator : RelationalOperator  Operator=<=
  Relational Operator1 : RelationalOperator  Operator=<=
  Sum1 : Sum  Inputs=|++
  Sum2 : Sum  Inputs=++|
  triangle_1 : Subsystem
  g21 : Outport
  g22 : Outport  Port=2
  tag scope: carry_g21=global
  wires:
  Sum1/1 -> Relational Operator/2
  Constant8/1 -> Sum2/2
  Sum2/1 -> Relational Operator1/1
  Data Type Conversion1/1 -> Gain1/1
  Constant7/1 -> Sum1/1
  triangle_1/1(carry_mod21) -> [carry_g21], Relational Operator1/2, Relational Operator/1
  Data Type Conversion/1 -> Gain/1
  Relational Operator1/1 -> Data Type Conversion1/1
  Relational Operator/1 -> Data Type Conversion/1
  m/1 -> Sum2/1, Sum1/2
  Gain/1 -> g21/1
  Gain1/1 -> g22/1

== system single_phase_multilevel/vi_ctrl/modulator3 ==
  m : Inport
  Constant7 : Constant  Value=-m_dead_time
  Constant8 : Constant  Value=m_dead_time
  Data Type Conversion : DataTypeConversion  OutDataTypeStr=double  SaturateOnIntegerOverflow=off  RndMeth=Floor
  Data Type Conversion1 : DataTypeConversion  OutDataTypeStr=double  SaturateOnIntegerOverflow=off  RndMeth=Floor
  Gain : Gain  Gain=Vgate_base
  Gain1 : Gain  Gain=Vgate_base
  Relational Operator : RelationalOperator  Operator=<=
  Relational Operator1 : RelationalOperator  Operator=<=
  Sum1 : Sum  Inputs=|++
  Sum2 : Sum  Inputs=++|
  triangle_1 : Subsystem
  g21 : Outport
  g22 : Outport  Port=2
  tag scope: carry_g31=global
  wires:
  m/1 -> Sum1/2, Sum2/1
  Relational Operator/1 -> Data Type Conversion/1
  Relational Operator1/1 -> Data Type Conversion1/1
  Data Type Conversion/1 -> Gain/1
  triangle_1/1(carry_mod21) -> Relational Operator/1, Relational Operator1/2, [carry_g31]
  Constant7/1 -> Sum1/1
  Data Type Conversion1/1 -> Gain1/1
  Sum2/1 -> Relational Operator1/1
  Constant8/1 -> Sum2/2
  Sum1/1 -> Relational Operator/2
  Gain/1 -> g21/1
  Gain1/1 -> g22/1

== system single_phase_multilevel/vi_ctrl/modulator4 ==
  m : Inport
  Constant7 : Constant  Value=-m_dead_time
  Constant8 : Constant  Value=m_dead_time
  Data Type Conversion : DataTypeConversion  OutDataTypeStr=double  SaturateOnIntegerOverflow=off  RndMeth=Floor
  Data Type Conversion1 : DataTypeConversion  OutDataTypeStr=double  SaturateOnIntegerOverflow=off  RndMeth=Floor
  Gain : Gain  Gain=Vgate_base
  Gain1 : Gain  Gain=Vgate_base
  Relational Operator : RelationalOperator  Operator=<=
  Relational Operator1 : RelationalOperator  Operator=<=
  Sum1 : Sum  Inputs=|++
  Sum2 : Sum  Inputs=++|
  triangle_1 : Subsystem
  g21 : Outport
  g22 : Outport  Port=2
  tag scope: carry_g41=global
  wires:
  m/1 -> Sum1/2, Sum2/1
  Relational Operator/1 -> Data Type Conversion/1
  Relational Operator1/1 -> Data Type Conversion1/1
  Data Type Conversion/1 -> Gain/1
  triangle_1/1(carry_mod21) -> Relational Operator/1, Relational Operator1/2, [carry_g41]
  Constant7/1 -> Sum1/1
  Data Type Conversion1/1 -> Gain1/1
  Sum2/1 -> Relational Operator1/1
  Constant8/1 -> Sum2/2
  Sum1/1 -> Relational Operator/2
  Gain/1 -> g21/1
  Gain1/1 -> g22/1

== system single_phase_multilevel/vi_ctrl/modulator5 ==
  m : Inport
  Constant7 : Constant  Value=-m_dead_time
  Constant8 : Constant  Value=m_dead_time
  Data Type Conversion : DataTypeConversion  OutDataTypeStr=double  SaturateOnIntegerOverflow=off  RndMeth=Floor
  Data Type Conversion1 : DataTypeConversion  OutDataTypeStr=double  SaturateOnIntegerOverflow=off  RndMeth=Floor
  Gain : Gain  Gain=Vgate_base
  Gain1 : Gain  Gain=Vgate_base
  Relational Operator : RelationalOperator  Operator=<=
  Relational Operator1 : RelationalOperator  Operator=<=
  Sum1 : Sum  Inputs=|++
  Sum2 : Sum  Inputs=++|
  triangle_1 : Subsystem
  g21 : Outport
  g22 : Outport  Port=2
  tag scope: carry_g51=global
  wires:
  Sum1/1 -> Relational Operator/2
  Constant8/1 -> Sum2/2
  Sum2/1 -> Relational Operator1/1
  Data Type Conversion1/1 -> Gain1/1
  Constant7/1 -> Sum1/1
  triangle_1/1(carry_mod21) -> [carry_g51], Relational Operator1/2, Relational Operator/1
  Data Type Conversion/1 -> Gain/1
  Relational Operator1/1 -> Data Type Conversion1/1
  Relational Operator/1 -> Data Type Conversion/1
  m/1 -> Sum2/1, Sum1/2
  Gain/1 -> g21/1
  Gain1/1 -> g22/1

== system single_phase_multilevel/vi_ctrl/pre-charge ==
  dm_in : Inport
  Ramp : simulink/Sources/Ramp  slope=-1  start=0  InitialOutput=0.5
  Saturation : Saturate  UpperLimit=0.25  LowerLimit=0
  Step1 : Step  Time=time_pwm_enable  SampleTime=0
  Switch : Switch  Criteria=u2 > Threshold  Threshold=0.5  SaturateOnIntegerOverflow=off  InputSameDT=off
  dm_out : Outport
  wires:
  Switch/1 -> dm_out/1
  ? -> Saturation/1
  Saturation/1 -> Switch/3
  dm_in/1 -> Switch/1
  Step1/1 -> Switch/2

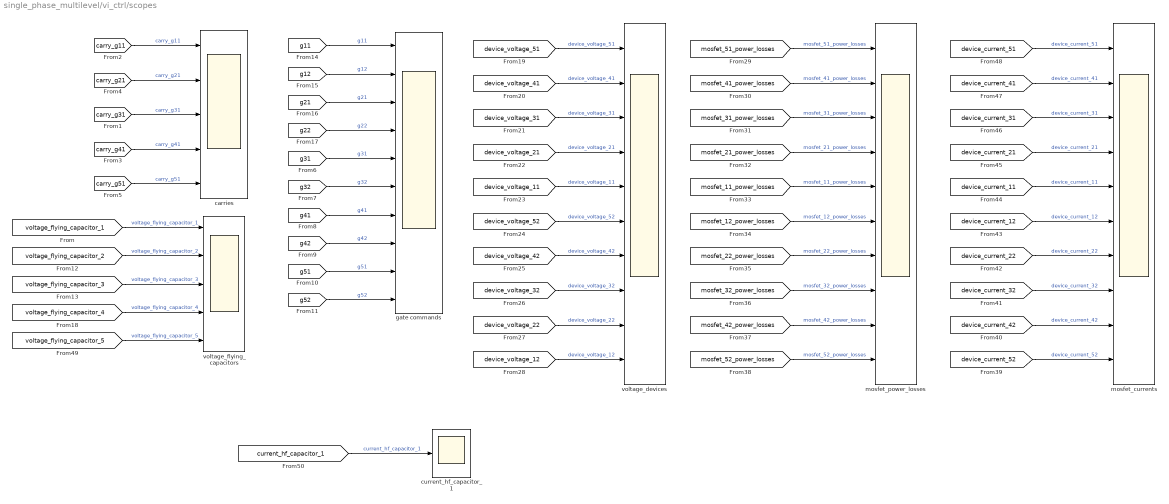
== system single_phase_multilevel/vi_ctrl/scopes ==
  carries : Scope  NumInputPorts=5
  current_hf_capacitor_1 : Scope
  gate commands : Scope  NumInputPorts=10
  mosfet_currents : Scope  NumInputPorts=10
  mosfet_power_losses : Scope  NumInputPorts=10
  voltage_devices : Scope  NumInputPorts=10
  voltage_flying_capacitors : Scope  NumInputPorts=5
  wires:
  [carry_g51] -> carries/5  "carry_g51"
  [g12] -> gate commands/2  "g12"
  [g11] -> gate commands/1  "g11"
  [g41] -> gate commands/7  "g41"
  [carry_g41] -> carries/4  "carry_g41"
  [g52] -> gate commands/10  "g52"
  [carry_g31] -> carries/3  "carry_g31"
  [g31] -> gate commands/5  "g31"
  [g21] -> gate commands/3  "g21"
  [voltage_flying_capacitor_4] -> voltage_flying_capacitors/4  "voltage_flying_capacitor_4"
  [carry_g11] -> carries/1  "carry_g11"
  [g42] -> gate commands/8  "g42"
  [voltage_flying_capacitor_1] -> voltage_flying_capacitors/1  "voltage_flying_capacitor_1"
  [g22] -> gate commands/4  "g22"
  [g32] -> gate commands/6  "g32"
  [g51] -> gate commands/9  "g51"
  [voltage_flying_capacitor_3] -> voltage_flying_capacitors/3  "voltage_flying_capacitor_3"
  [voltage_flying_capacitor_2] -> voltage_flying_capacitors/2  "voltage_flying_capacitor_2"
  [carry_g21] -> carries/2  "carry_g21"
  [device_current_11] -> mosfet_currents/5  "device_current_11"
  [mosfet_12_power_losses] -> mosfet_power_losses/6  "mosfet_12_power_losses"
  [device_current_32] -> mosfet_currents/8  "device_current_32"
  [mosfet_21_power_losses] -> mosfet_power_losses/4  "mosfet_21_power_losses"
  [device_voltage_42] -> voltage_devices/7  "device_voltage_42"
  [device_voltage_21] -> voltage_devices/4  "device_voltage_21"
  [device_current_12] -> mosfet_currents/6  "device_current_12"
  [device_voltage_52] -> voltage_devices/6  "device_voltage_52"
  [device_voltage_41] -> voltage_devices/2  "device_voltage_41"
  [device_voltage_51] -> voltage_devices/1  "device_voltage_51"
  [device_voltage_11] -> voltage_devices/5  "device_voltage_11"
  [mosfet_31_power_losses] -> mosfet_power_losses/3  "mosfet_31_power_losses"
  [device_voltage_22] -> voltage_devices/9  "device_voltage_22"
  [device_current_51] -> mosfet_currents/1  "device_current_51"
  [device_current_41] -> mosfet_currents/2  "device_current_41"
  [device_voltage_12] -> voltage_devices/10  "device_voltage_12"
  [device_voltage_32] -> voltage_devices/8  "device_voltage_32"
  [device_voltage_31] -> voltage_devices/3  "device_voltage_31"
  [mosfet_32_power_losses] -> mosfet_power_losses/8  "mosfet_32_power_losses"
  [mosfet_11_power_losses] -> mosfet_power_losses/5  "mosfet_11_power_losses"
  [mosfet_51_power_losses] -> mosfet_power_losses/1  "mosfet_51_power_losses"
  [mosfet_41_power_losses] -> mosfet_power_losses/2  "mosfet_41_power_losses"
  [mosfet_42_power_losses] -> mosfet_power_losses/9  "mosfet_42_power_losses"
  [mosfet_52_power_losses] -> mosfet_power_losses/10  "mosfet_52_power_losses"
  [mosfet_22_power_losses] -> mosfet_power_losses/7  "mosfet_22_power_losses"
  [device_current_42] -> mosfet_currents/9  "device_current_42"
  [device_current_31] -> mosfet_currents/3  "device_current_31"
  [device_current_22] -> mosfet_currents/7  "device_current_22"
  [device_current_21] -> mosfet_currents/4  "device_current_21"
  [device_current_52] -> mosfet_currents/10  "device_current_52"
  [voltage_flying_capacitor_5] -> voltage_flying_capacitors/5  "voltage_flying_capacitor_5"
  [current_hf_capacitor_1] -> current_hf_capacitor_1/1  "current_hf_capacitor_1"

== system single_phase_multilevel/vi_ctrl/single_phase_contrl_system ==
  1/Ti2 : Gain  Gain=1/V_FS  SaturateOnIntegerOverflow=on  OutDataTypeStr=Inherit: Same as input  ParamDataTypeStr=Inherit: Same as input
  Constant1 : Constant  Value=0
  Math Function : Math  Operator=magnitude^2
  Math Function1 : Math  Operator=magnitude^2
  Sqrt : Sqrt
  Sum1 : Sum  Inputs=|-+
  Sum2 : Sum  Inputs=+-|
  Sum3 : Sum  Inputs=|++
  Sum4 : Sum  Inputs=|-+
  Zero-Order Hold4 : ZeroOrderHold  SampleTime=ts
  acquisition_and_scaling_current : Subsystem
  acquisition_and_scaling_voltage : Subsystem
  alpha_beta_transformation_i : Subsystem
  alpha_beta_transformation_v : Subsystem
  alphabeta2dq : Subsystem
  dq2alphabeta : Subsystem
  i_alpha_beta : Scope  NumInputPorts=2
  idq : Scope  NumInputPorts=2
  inverter current/voltage : Scope  NumInputPorts=3
  phase_gen : Subsystem
  pi_d : Subsystem
  pi_q : Subsystem
  pi_v : Subsystem
  reference_flt : Subsystem
  v_reference : Step  Time=precharge_off  After=230*sqrt(2)  SampleTime=0
  alpha : Outport
  tag scope: uout_magnitude_pu=global, uout_magnitude_pu_ref=global
  wires:
  [inverter_current_output] -> inverter current/voltage/1  "inverter_current_output_modA"
  [inverter_current_output] -> acquisition_and_scaling_current/1(in)
  pi_d/1(Vd_out) -> dq2alphabeta/1(d)
  pi_v/1(i_ref_internal) -> Sum2/1
  Zero-Order Hold4/1 -> reference_flt/1(input)
  alpha_beta_transformation_v/2(beta) -> Math Function1/1
  [inverter_voltage_output] -> inverter current/voltage/2  "inverter_voltager_output_modA"
  alphabeta2dq/2("q ") -> idq/2, Sum1/1
  dq2alphabeta/1(alpha) -> alpha/1
  [inverter_voltage_output] -> acquisition_and_scaling_voltage/1(in)
  Constant1/1 -> Sum1/2
  alphabeta2dq/1("d ") -> idq/1, Sum2/2
  v_reference/1 -> 1/Ti2/1
  Sum4/1 -> pi_v/1(e)
  Math Function1/1 -> Sum3/2
  phase_gen/1(theta) -> alphabeta2dq/3(wt), dq2alphabeta/3(wt)
  1/Ti2/1 -> Zero-Order Hold4/1
  acquisition_and_scaling_current/1(out) -> alpha_beta_transformation_i/1(in)
  Sum3/1 -> Sqrt/1
  Sum1/1 -> pi_q/1(iq_tilde)
  Math Function/1 -> Sum3/1
  Sqrt/1 -> [uout_magnitude_pu], Sum4/1
  pi_q/1(Vd_out) -> dq2alphabeta/2(q)
  Sum2/1 -> pi_d/1(id_tilde)
  alpha_beta_transformation_i/1(alpha) -> i_alpha_beta/1, alphabeta2dq/1(alpha)
  alpha_beta_transformation_i/2(beta) -> i_alpha_beta/2, alphabeta2dq/2(beta)
  acquisition_and_scaling_voltage/1(out) -> alpha_beta_transformation_v/1(in)
  alpha_beta_transformation_v/1(alpha) -> Math Function/1
  [inverter_current_stack] -> inverter current/voltage/3  "inverter_current_stack_modA"
  reference_flt/1(output) -> [uout_magnitude_pu_ref], Sum4/2

== system single_phase_multilevel/flying_capacitor_leg/switch_11/gate_driver ==
  cmd : Inport
  Controlled Voltage Source : fl_lib/Electrical/Electrical Sources/Controlled Voltage Source
  Diode1 : fl_lib/Electrical/Electrical Elements/Diode  Vf=0.6 V  Ron=0.3 Ohm  Goff=1e-8 1/Ohm  i_specify=off  i_priority=None  i=0 A  i_nominal_specify=off  i_nominal_unit=A  i_nominal_value=1  v_specify=off  v_priority=None  v=0 V  v_nominal_specify=off  v_nominal_unit=V  v_nominal_value=1
  Diode2 : fl_lib/Electrical/Electrical Elements/Diode  Vf=0.6 V  Ron=0.3 Ohm  Goff=1e-8 1/Ohm  i_specify=off  i_priority=None  i=0 A  i_nominal_specify=off  i_nominal_unit=A  i_nominal_value=1  v_specify=off  v_priority=None  v=0 V  v_nominal_specify=off  v_nominal_unit=V  v_nominal_value=1
  Resistor : fl_lib/Electrical/Electrical Elements/Resistor  R=Rg_on Ohm  i_specify=off  i_priority=None  i=0 A  i_nominal_specify=off  i_nominal_unit=A  i_nominal_value=1  v_specify=off  v_priority=None  v=0 V  v_nominal_specify=off  v_nominal_unit=V  v_nominal_value=1
  Resistor1 : fl_lib/Electrical/Electrical Elements/Resistor  R=Rg_off Ohm  i_specify=off  i_priority=None  i=0 A  i_nominal_specify=off  i_nominal_unit=A  i_nominal_value=1  v_specify=off  v_priority=None  v=0 V  v_nominal_specify=off  v_nominal_unit=V  v_nominal_value=1
  Simulink-PS Converter : nesl_utility/Simulink-PS Converter  PhysicalDomain=network_engine_domain  SubClassName=ps_input  LeftPortType=input  RightPortType=output  PseudoPeriodic=off  Frequencies=[]  NoiseDistribution=none  NoiseParameters=[]  Unit=V  AffineConversion=off  FilteringAndDerivatives=provide  SimscapeFilterOrder=1  InputFilterTimeConstant=0.001  UdotUserProvided=0
  gate : PMIOPort  Side=Right
  source : PMIOPort  Port=2  Side=Right
  wires:
  cmd/1 -> Simulink-PS Converter/1
  connections:
  Resistor/LConn1 -- Controlled Voltage Source/LConn1 -- Resistor1/LConn1
  Diode2/LConn1 -- Resistor/RConn1
  Controlled Voltage Source/RConn1 -- Simulink-PS Converter/RConn1
  Controlled Voltage Source/RConn2 -- source/RConn1
  Diode1/LConn1 -- gate/RConn1 -- Diode2/RConn1
  Diode1/RConn1 -- Resistor1/RConn1

== system single_phase_multilevel/flying_capacitor_leg/switch_12/gate_driver ==
  cmd : Inport
  Controlled Voltage Source : fl_lib/Electrical/Electrical Sources/Controlled Voltage Source
  Diode1 : fl_lib/Electrical/Electrical Elements/Diode  Vf=0.6 V  Ron=0.3 Ohm  Goff=1e-8 1/Ohm  i_specify=off  i_priority=None  i=0 A  i_nominal_specify=off  i_nominal_unit=A  i_nominal_value=1  v_specify=off  v_priority=None  v=0 V  v_nominal_specify=off  v_nominal_unit=V  v_nominal_value=1
  Diode2 : fl_lib/Electrical/Electrical Elements/Diode  Vf=0.6 V  Ron=0.3 Ohm  Goff=1e-8 1/Ohm  i_specify=off  i_priority=None  i=0 A  i_nominal_specify=off  i_nominal_unit=A  i_nominal_value=1  v_specify=off  v_priority=None  v=0 V  v_nominal_specify=off  v_nominal_unit=V  v_nominal_value=1
  Resistor : fl_lib/Electrical/Electrical Elements/Resistor  R=Rg_on Ohm  i_specify=off  i_priority=None  i=0 A  i_nominal_specify=off  i_nominal_unit=A  i_nominal_value=1  v_specify=off  v_priority=None  v=0 V  v_nominal_specify=off  v_nominal_unit=V  v_nominal_value=1
  Resistor1 : fl_lib/Electrical/Electrical Elements/Resistor  R=Rg_off Ohm  i_specify=off  i_priority=None  i=0 A  i_nominal_specify=off  i_nominal_unit=A  i_nominal_value=1  v_specify=off  v_priority=None  v=0 V  v_nominal_specify=off  v_nominal_unit=V  v_nominal_value=1
  Simulink-PS Converter : nesl_utility/Simulink-PS Converter  PhysicalDomain=network_engine_domain  SubClassName=ps_input  LeftPortType=input  RightPortType=output  PseudoPeriodic=off  Frequencies=[]  NoiseDistribution=none  NoiseParameters=[]  Unit=V  AffineConversion=off  FilteringAndDerivatives=provide  SimscapeFilterOrder=1  InputFilterTimeConstant=0.001  UdotUserProvided=0
  gate : PMIOPort  Side=Right
  source : PMIOPort  Port=2  Side=Right
  wires:
  cmd/1 -> Simulink-PS Converter/1
  connections:
  Resistor/LConn1 -- Controlled Voltage Source/LConn1 -- Resistor1/LConn1
  Diode2/LConn1 -- Resistor/RConn1
  Controlled Voltage Source/RConn1 -- Simulink-PS Converter/RConn1
  Controlled Voltage Source/RConn2 -- source/RConn1
  Diode1/LConn1 -- gate/RConn1 -- Diode2/RConn1
  Diode1/RConn1 -- Resistor1/RConn1

== system single_phase_multilevel/flying_capacitor_leg/switch_21/gate_driver ==
  cmd : Inport
  Controlled Voltage Source : fl_lib/Electrical/Electrical Sources/Controlled Voltage Source
  Diode1 : fl_lib/Electrical/Electrical Elements/Diode  Vf=0.6 V  Ron=0.3 Ohm  Goff=1e-8 1/Ohm  i_specify=off  i_priority=None  i=0 A  i_nominal_specify=off  i_nominal_unit=A  i_nominal_value=1  v_specify=off  v_priority=None  v=0 V  v_nominal_specify=off  v_nominal_unit=V  v_nominal_value=1
  Diode2 : fl_lib/Electrical/Electrical Elements/Diode  Vf=0.6 V  Ron=0.3 Ohm  Goff=1e-8 1/Ohm  i_specify=off  i_priority=None  i=0 A  i_nominal_specify=off  i_nominal_unit=A  i_nominal_value=1  v_specify=off  v_priority=None  v=0 V  v_nominal_specify=off  v_nominal_unit=V  v_nominal_value=1
  Resistor : fl_lib/Electrical/Electrical Elements/Resistor  R=Rg_on Ohm  i_specify=off  i_priority=None  i=0 A  i_nominal_specify=off  i_nominal_unit=A  i_nominal_value=1  v_specify=off  v_priority=None  v=0 V  v_nominal_specify=off  v_nominal_unit=V  v_nominal_value=1
  Resistor1 : fl_lib/Electrical/Electrical Elements/Resistor  R=Rg_off Ohm  i_specify=off  i_priority=None  i=0 A  i_nominal_specify=off  i_nominal_unit=A  i_nominal_value=1  v_specify=off  v_priority=None  v=0 V  v_nominal_specify=off  v_nominal_unit=V  v_nominal_value=1
  Simulink-PS Converter : nesl_utility/Simulink-PS Converter  PhysicalDomain=network_engine_domain  SubClassName=ps_input  LeftPortType=input  RightPortType=output  PseudoPeriodic=off  Frequencies=[]  NoiseDistribution=none  NoiseParameters=[]  Unit=V  AffineConversion=off  FilteringAndDerivatives=provide  SimscapeFilterOrder=1  InputFilterTimeConstant=0.001  UdotUserProvided=0
  gate : PMIOPort  Side=Right
  source : PMIOPort  Port=2  Side=Right
  wires:
  cmd/1 -> Simulink-PS Converter/1
  connections:
  Resistor/LConn1 -- Controlled Voltage Source/LConn1 -- Resistor1/LConn1
  Diode2/LConn1 -- Resistor/RConn1
  Controlled Voltage Source/RConn1 -- Simulink-PS Converter/RConn1
  Controlled Voltage Source/RConn2 -- source/RConn1
  Diode1/LConn1 -- gate/RConn1 -- Diode2/RConn1
  Diode1/RConn1 -- Resistor1/RConn1

== system single_phase_multilevel/flying_capacitor_leg/switch_22/gate_driver ==
  cmd : Inport
  Controlled Voltage Source : fl_lib/Electrical/Electrical Sources/Controlled Voltage Source
  Diode1 : fl_lib/Electrical/Electrical Elements/Diode  Vf=0.6 V  Ron=0.3 Ohm  Goff=1e-8 1/Ohm  i_specify=off  i_priority=None  i=0 A  i_nominal_specify=off  i_nominal_unit=A  i_nominal_value=1  v_specify=off  v_priority=None  v=0 V  v_nominal_specify=off  v_nominal_unit=V  v_nominal_value=1
  Diode2 : fl_lib/Electrical/Electrical Elements/Diode  Vf=0.6 V  Ron=0.3 Ohm  Goff=1e-8 1/Ohm  i_specify=off  i_priority=None  i=0 A  i_nominal_specify=off  i_nominal_unit=A  i_nominal_value=1  v_specify=off  v_priority=None  v=0 V  v_nominal_specify=off  v_nominal_unit=V  v_nominal_value=1
  Resistor : fl_lib/Electrical/Electrical Elements/Resistor  R=Rg_on Ohm  i_specify=off  i_priority=None  i=0 A  i_nominal_specify=off  i_nominal_unit=A  i_nominal_value=1  v_specify=off  v_priority=None  v=0 V  v_nominal_specify=off  v_nominal_unit=V  v_nominal_value=1
  Resistor1 : fl_lib/Electrical/Electrical Elements/Resistor  R=Rg_off Ohm  i_specify=off  i_priority=None  i=0 A  i_nominal_specify=off  i_nominal_unit=A  i_nominal_value=1  v_specify=off  v_priority=None  v=0 V  v_nominal_specify=off  v_nominal_unit=V  v_nominal_value=1
  Simulink-PS Converter : nesl_utility/Simulink-PS Converter  PhysicalDomain=network_engine_domain  SubClassName=ps_input  LeftPortType=input  RightPortType=output  PseudoPeriodic=off  Frequencies=[]  NoiseDistribution=none  NoiseParameters=[]  Unit=V  AffineConversion=off  FilteringAndDerivatives=provide  SimscapeFilterOrder=1  InputFilterTimeConstant=0.001  UdotUserProvided=0
  gate : PMIOPort  Side=Right
  source : PMIOPort  Port=2  Side=Right
  wires:
  cmd/1 -> Simulink-PS Converter/1
  connections:
  Resistor/LConn1 -- Controlled Voltage Source/LConn1 -- Resistor1/LConn1
  Diode2/LConn1 -- Resistor/RConn1
  Controlled Voltage Source/RConn1 -- Simulink-PS Converter/RConn1
  Controlled Voltage Source/RConn2 -- source/RConn1
  Diode1/LConn1 -- gate/RConn1 -- Diode2/RConn1
  Diode1/RConn1 -- Resistor1/RConn1
